simulink model "myfuzzylogic"  (R2014a)
settings: Solver=FixedStepDiscrete  StartTime=0.0  StopTime=inf  FixedStep=0.01  RelTol=1e-3
values from neighbouring files (symbols this model uses):
  matrix = readfis('fuzzyPID.fis')    [fuzzy.m]
libraries: fuzblock x1
settings Model: Creator=Administrator  LastModifiedBy=Administrator
settings OptimizationCC: InlineParams=on  UseSpecifiedMinMax=on  InlineInvariantSignals=on  ZeroExternalMemoryAtStartup=off  ZeroInternalMemoryAtStartup=off  NoFixptDivByZeroProtection=on  EfficientFloat2IntCast=on  OptimizeModelRefInitCode=on  LifeSpan=Inf
settings HardwareCC: ProdBitPerInt=16  ProdBitPerPointer=16  ProdIntDivRoundTo=Zero  ProdEndianess=LittleEndian  ProdWordSize=16  ProdHWDeviceType=STMicroelectronics->ST10/Super10
settings RTWCC: SystemTargetFile=ert.tlc  TemplateMakefile=ert_default_tmf  Description=Embedded Coder  GenerateReport=on  ProcessScript=ert_make_rtw_hook  IncludeHyperlinkInReport=on  LaunchReport=on
settings CodeAppCC: IgnoreCustomStorageClasses=off
settings ERTTargetCC: UtilityFuncGeneration=Shared location  ParMdlRefBuildCompliant=on  CompOptLevelCompliant=on  ConcurrentExecutionCompliant=on  IncludeMdlTerminateFcn=off  CombineSignalStateStructs=on  SuppressErrorStatus=on  ERTFirstTimeCompliant=on  SupportNonFinite=off  ModelStepFunctionPrototypeControlCompliant=on  CPPClassGenCompliant=on  InlinedParameterPlacement=Hierarchical  ERTCustomFileTemplate=example_file_process.tlc  ConvertIfToSwitch=on  SuppressUnreachableDefaultCases=on

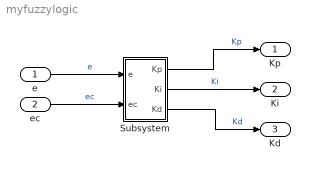
== system myfuzzylogic ==
  e : Inport
  ec : Inport  Port=2
  Subsystem : Subsystem
  Kp : Outport
  Ki : Outport  Port=2
  Kd : Outport  Port=3
  wires:
  e/1 -> Subsystem/1(e)  "e"
  ec/1 -> Subsystem/2(ec)  "ec"
  Subsystem/1(Kp) -> Kp/1  "Kp"
  Subsystem/2(Ki) -> Ki/1  "Ki"
  Subsystem/3(Kd) -> Kd/1  "Kd"

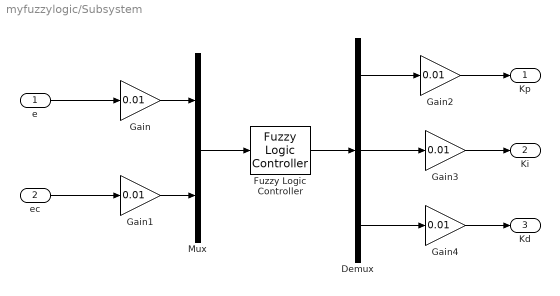
== system myfuzzylogic/Subsystem ==
  e : Inport
  ec : Inport  Port=2
  Demux : Demux  Outputs=3
  Fuzzy Logic Controller : fuzblock/Fuzzy Logic  Controller  fis=[matrix]
  Gain{,1..4} (5 alike) : Gain  Gain=0.01
  Mux : Mux  Inputs=2
  Kp : Outport
  Ki : Outport  Port=2
  Kd : Outport  Port=3
  wires:
  e/1 -> Gain/1
  Gain1/1 -> Mux/2
  Gain/1 -> Mux/1
  ec/1 -> Gain1/1
  Fuzzy Logic Controller/1 -> Demux/1
  Gain4/1 -> Kd/1
  Gain2/1 -> Kp/1
  Mux/1 -> Fuzzy Logic Controller/1
  Gain3/1 -> Ki/1
  Demux/2 -> Gain3/1
  Demux/1 -> Gain2/1
  Demux/3 -> Gain4/1
